simulink model "test3a"  (R2014b)
settings: Solver=FixedStepDiscrete  StartTime=0.0  StopTime=100  RelTol=1e-3
libraries: dspsrcs4 x1, dspsnks4 x1
settings Model: CovMetricSettings=d  Creator=The MathWorks Inc.  LastModifiedBy=Theo
settings DataIOCC: SignalLoggingSaveFormat=ModelDataLogs  SignalLoggingName=sigsOut
settings OptimizationCC: BlockReduction=off  BooleanDataType=off  ExpressionDepthLimit=2147483647  EfficientMapNaN2IntZero=off
settings DebuggingCC: SaveWithParameterizedLinksMsg=none  UnderspecifiedInitializationDetection=Classic  MergeDetectMultiDrivingBlocksExec=none  SignalResolutionControl=TryResolveAllWithWarning  SolverPrmCheckMsg=none  MultiTaskDSMMsg=warning  MultiTaskCondExecSysMsg=none  FcnCallInpInsideContextMsg=UseLocalSettings  StateNameClashWarn=warning
settings HardwareCC: TargetUnknown=on
settings RTWCC: IncludeERTFirstTime=on
settings GRTTargetCC: CombineOutputUpdateFcns=off  GRTInterface=on

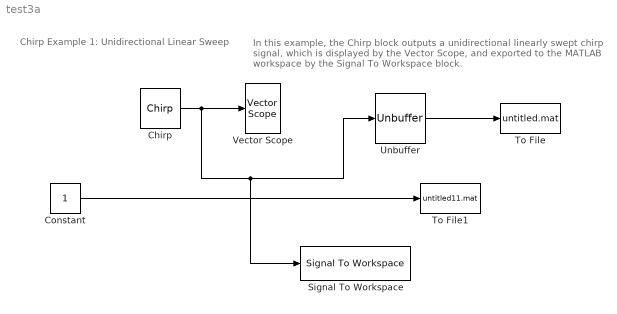
== system test3a ==
  note: Chirp Example 1:
      | Unidirectional Linear Sweep
  note: In this example, the Chirp block outputs a unidirectional linearly swept
      | chirp signal, which is displayed by the Vector Scope, and exported to
      | the MATLAB workspace by the Signal To Workspace block.
  Chirp : dspsrcs4/Chirp  sweep=Linear  mode=Unidirectional  f0=1  f1=250  t1=10  Tsweep=10  phase=0  Ts=1/4096  spf=400  datatype=Double
  Constant : Constant
  Signal To Workspace : SignalToWorkspace  VariableName=dsp_examples_yout
      settings: CopyFcn=dspblkcopystw(gcbh);  Decimation=2
  To File : ToFile
  To File1 : ToFile  Filename=untitled11.mat  SaveFormat=Timeseries
  Unbuffer : Unbuffer  SampleBasedProcessing=Same as frame based
  Vector Scope : dspsnks4/Vector Scope  ScopeProperties=on  Domain=Time  HorizSpan=50  DisplayProperties=off  AxisGrid=on  Memory=off  FrameNumber=on  AxisLegend=off  AxisZoom=off  OpenScopeAtSimStart=on  OpenScopeImmediately=off  FigPos=[720 450 650 320]  AxisProperties=off  XUnits=Hertz  XRange=[0...Fs/2]  InheritXIncr=on  XIncr=1  XLabel=Time  XLimit=Auto  XMin=0  XMax=1  XStart=0  YUnits=dB  YLabel=Amplitude  LineProperties=off  XAxisParamsVer=6.9
      settings: YMin=-10  YMax=10
  wires:
  Chirp/1 -> Unbuffer/1, Signal To Workspace/1, Vector Scope/1
  Constant/1 -> To File1/1
  Unbuffer/1 -> To File/1
